simulink model "Task3"  (R2015b)
settings: Solver=FixedStepDiscrete  StartTime=0.0  StopTime=10.0  FixedStep=0.0001  RelTol=1e-3
undefined symbols (not defined in the file or in its folder): A, B, C
libraries: simulink x1
settings Model: Creator=User  LastModifiedBy=User

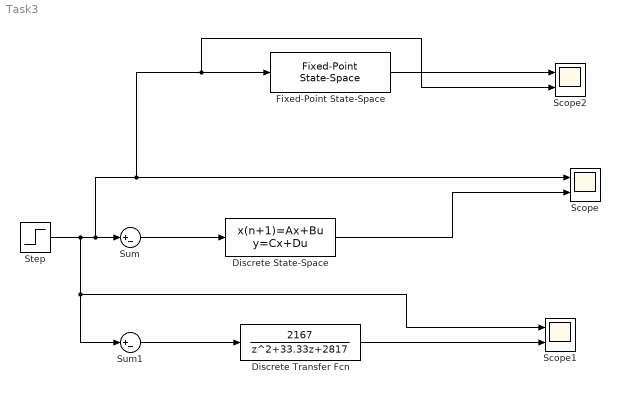
== system Task3 ==
  Discrete Transfer Fcn : DiscreteTransferFcn  Numerator=[2167]  Denominator=[1 33.33 2817]  SampleTime=0.0001
  Discrete State-Space : DiscreteStateSpace  A=A  B=B  C=C  D=0  SampleTime=0.0001
  Fixed-Point State-Space : simulink/Additional Math & Discrete/Additional Discrete/Fixed-Point State-Space  A=A  B=B  C=C  D=[0]  X0=0.0001  InternalDataType=fixdt('double')  StateEqScaling=2^0  OutputEqScaling=2^0  DoSatur=off
  Scope : Scope  NumInputPorts=2
  Scope1 : Scope  NumInputPorts=2
  Scope2 : Scope  NumInputPorts=2
  Step : Step  SampleTime=0.0001
  Sum : Sum  Inputs=|+-
  Sum1 : Sum  Inputs=|+-
  wires:
  Discrete State-Space/1 -> Scope/2
  Sum/1 -> Discrete State-Space/1
  Step/1 -> Sum1/1, Scope1/1, Scope2/2, Fixed-Point State-Space/1, Scope/1, Sum/1
  Discrete Transfer Fcn/1 -> Scope1/2
  Sum1/1 -> Discrete Transfer Fcn/1
  Fixed-Point State-Space/1 -> Scope2/1
